simulink model "lateral_autopilot"  (R2016b)
settings: Solver=VariableStepAuto  StartTime=0.0  StopTime=t_end  RelTol=1e-3
values from neighbouring files (symbols this model uses):
  a_phi_1 = 2.87    [parameters_longitudal_autopilot.m]
  a_phi_2 = -0.65    [parameters_longitudal_autopilot.m]
  chi_c = 10*deg2rad    [run_task_2e.m]    (also in run_task_2f.m)
  d = 8*deg2rad    [run_task_2e.m]    (also in run_task_2f.m)
  delta_a_max = 25*deg2rad    (= 0.436332312999)    [parameters_longitudal_autopilot.m]
  g = 9.81    [parameters_longitudal_autopilot.m]
  k_d_phi = (2*zeta_phi*omega_n_phi - a_phi_1) / a_phi_2    [parameters_longitudal_autopilot.m]
  k_i_chi = omega_n_chi^2*V_g/g    [parameters_longitudal_autopilot.m]    (also in regulation_parameters_2_2.m)
  k_i_phi = -1    [parameters_longitudal_autopilot.m]
  k_p_chi = 2*zeta_chi*omega_n_chi*V_g/g    [parameters_longitudal_autopilot.m]    (also in regulation_parameters_2_2.m)
  k_p_phi = sgn(a_phi_2)*delta_a_max /e_phi_max    [parameters_longitudal_autopilot.m]
  V_g = 637/3.6    (= 176.944444444)    [parameters_longitudal_autopilot.m]
settings Model: Creator=Alexandra  LastModifiedBy=Alexandra

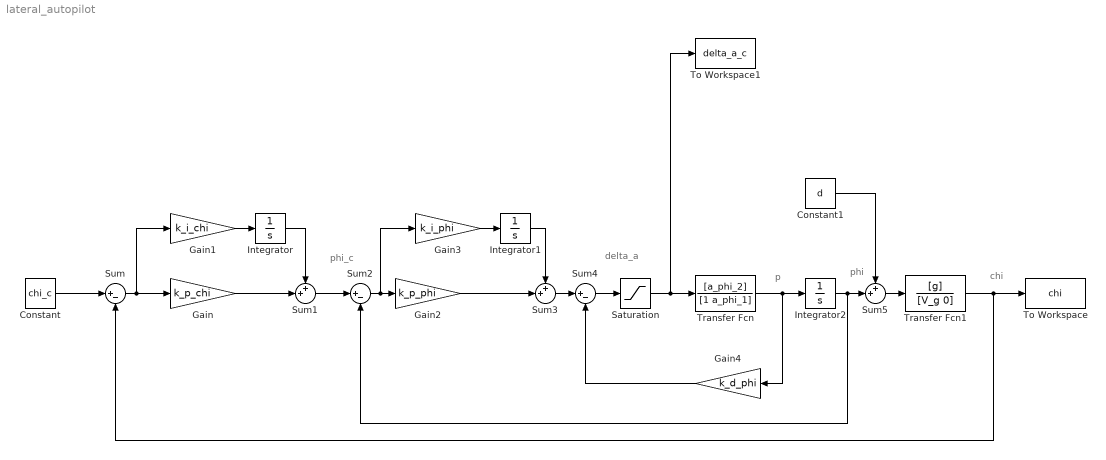
== system lateral_autopilot ==
  note: phi_c
  note: delta_a
  note: phi
  note: chi
  note: p
  Constant : Constant  Value=chi_c
  Constant1 : Constant  Value=d
  Gain : Gain  Gain=k_p_chi
  Gain1 : Gain  Gain=k_i_chi
  Gain2 : Gain  Gain=k_p_phi
  Gain3 : Gain  Gain=k_i_phi
  Gain4 : Gain  Gain=k_d_phi
  Integrator : Integrator
  Integrator1 : Integrator
  Integrator2 : Integrator
  Saturation : Saturate  UpperLimit=delta_a_max  LowerLimit=-delta_a_max
  Sum : Sum  Inputs=|+-
  Sum1 : Sum  Inputs=++|
  Sum2 : Sum  Inputs=|+-
  Sum3 : Sum  Inputs=++|
  Sum4 : Sum  Inputs=|+-
  Sum5 : Sum  Inputs=++|
  To Workspace : ToWorkspace  VariableName=chi  SaveFormat=Structure With Time  SampleTime=-1
  To Workspace1 : ToWorkspace  VariableName=delta_a_c  SaveFormat=Structure With Time  SampleTime=-1
  Transfer Fcn : TransferFcn  Numerator=[a_phi_2]  Denominator=[1 a_phi_1]
  Transfer Fcn1 : TransferFcn  Numerator=[g]  Denominator=[V_g 0]
  wires:
  Constant/1 -> Sum/1
  Sum/1 -> Gain1/1, Gain/1
  Gain1/1 -> Integrator/1
  Gain/1 -> Sum1/2
  Integrator/1 -> Sum1/1
  Sum1/1 -> Sum2/1
  Sum2/1 -> Gain3/1, Gain2/1
  Gain3/1 -> Integrator1/1
  Integrator1/1 -> Sum3/1
  Gain2/1 -> Sum3/2
  Sum3/1 -> Sum4/1
  Transfer Fcn/1 -> Gain4/1, Integrator2/1
  Integrator2/1 -> Sum2/2, Sum5/2
  Gain4/1 -> Sum4/2
  Constant1/1 -> Sum5/1
  Sum5/1 -> Transfer Fcn1/1
  Transfer Fcn1/1 -> To Workspace/1, Sum/2
  Sum4/1 -> Saturation/1
  Saturation/1 -> To Workspace1/1, Transfer Fcn/1
